simulink model "A3_Greenhouse_Temperature_Control_OnOff_Heater - Copy"  (R2020a)
settings: Solver=VariableStepAuto  StartTime=0.0  StopTime=30000  RelTol=1e-3
settings Model: Creator=mitch  LastModifiedBy=mitch

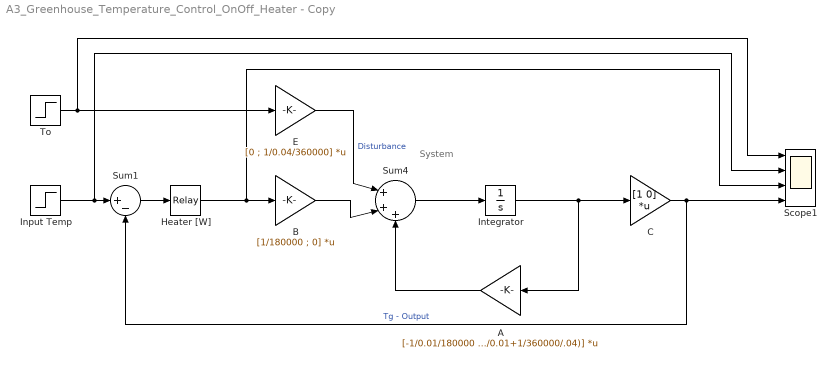
== system A3_Greenhouse_Temperature_Control_OnOff_Heater - Copy ==
  note: System
  A : Gain  Gain=[-1/0.01/180000 1/0.01/180000; 1/360000/0.01 -(1/360000/0.01+1/360000/.04)]  Multiplication=Matrix(K*u)
  B : Gain  Gain=[1/180000 ; 0]  Multiplication=Matrix(K*u)
  C : Gain  Gain=[1 0]  Multiplication=Matrix(K*u)
  E : Gain  Gain=[0 ; 1/0.04/360000]  Multiplication=Matrix(K*u)
  "Heater [W] " : Relay  OnSwitchValue=2  OffSwitchValue=-2  OnOutputValue=1500
  Input Temp : Step  Time=5000  Before=10  After=15  SampleTime=0
  Integrator : Integrator  InitialCondition=[10; 0]  LimitOutput=on  UpperSaturationLimit=20
  Scope1 : Scope  NumInputPorts=4
  Sum1 : Sum  Inputs=|+-
  Sum4 : Sum  Inputs=|+++
  To : Step  Time=15000  After=-10  SampleTime=0
  wires:
  B/1 -> Sum4/2
  To/1 -> E/1, Scope1/1
  E/1 -> Sum4/1  "Disturbance"
  Sum4/1 -> Integrator/1
  Integrator/1 -> C/1, A/1
  A/1 -> Sum4/3
  C/1 -> Sum1/2, Scope1/4  "Tg - Output"
  Input Temp/1 -> Scope1/2, Sum1/1
  Sum1/1 -> "Heater [W] "/1
  "Heater [W] "/1 -> Scope1/3, B/1
